simulink model "EKF_SIL_02_newdelIpsOOSM"  (R2015a)
settings: Solver=ode45  StartTime=0.0  StopTime=50  RelTol=1e-3
model workspace: external: MATLAB File InitOOSM.m (data not in the file)
values from neighbouring files (symbols this model uses):
  Cov_nu = [0.005 0 0 0 ... (first row only)    [InitOOSM.m]    (also in InitSIL.m; Init_Model_02_Simulink.m; Init_Model_02_Simulink_SIL1.m)
  Cov_r = [0.003 0 0 ... (first row only)    [InitOOSM.m]    (also in InitSIL.m; Init_Model_02_Simulink.m; Init_Model_02_Simulink_SIL1.m)
  e_force_x = 0    [InitOOSM.m]    (also in InitSIL.m; Init_Model_02_Simulink.m; Init_Model_02_Simulink_SIL1.m)
  e_force_y = 0    [InitOOSM.m]    (also in InitSIL.m; Init_Model_02_Simulink.m; Init_Model_02_Simulink_SIL1.m)
  e_force_z = 0    [InitOOSM.m]    (also in InitSIL.m; Init_Model_02_Simulink.m; Init_Model_02_Simulink_SIL1.m)
  ieps = [-0.7071;0;0;0.7071]    [InitOOSM.m]    (also in InitSIL.m; Init_Model_02_Simulink.m = [-0.7071; 0; 0; 0.7071]; Init_Model_02_Simulink_SIL1.m)
  ita = [0.5;0.5;0.5;0.5]    [InitOOSM.m]    (also in InitSIL.m; Init_Model_02_Simulink.m = [0.5; 0.5; 0.5; 0.5]; Init_Model_02_Simulink_SIL1.m)
  n = 0.00    (= 0)    [InitOOSM.m]    (also in InitSIL.m; Init_Model_02_Simulink.m; Init_Model_02_Simulink_SIL1.m)
  P_0 = 0.5*eye(18,18)    [InitOOSM.m]    (also in InitSIL.m = 0.05*eye(12,12); Init_Model_02_Simulink.m = 0.005*eye(12,12); Init_Model_02_Simulink_SIL1.m = 0.005*eye(12,12))
  P_k = Simulink.Signal    [InitOOSM.m]    (also in InitSIL.m; Init_Model_02_Simulink.m; Init_Model_02_Simulink_SIL1.m)
  p_x = 0.75    [InitOOSM.m]    (also in InitSIL.m; Init_Model_02_Simulink.m; Init_Model_02_Simulink_SIL1.m)
  p_y = 0.125    [InitOOSM.m]    (also in InitSIL.m; Init_Model_02_Simulink.m; Init_Model_02_Simulink_SIL1.m)
  p_z = -0.8    [InitOOSM.m]    (also in InitSIL.m; Init_Model_02_Simulink.m; Init_Model_02_Simulink_SIL1.m)
  parameter_gravitation = 3.986005E+14    (= 398600500000000)    [InitOOSM.m]    (also in InitSIL.m; Init_Model_02_Simulink.m; Init_Model_02_Simulink_SIL1.m)
  rho = [0.04;0;0.3]    [InitOOSM.m]    (also in InitSIL.m; Init_Model_02_Simulink.m = [0.04; 0; 0.3]; Init_Model_02_Simulink_SIL1.m)
  rho_c = [-0.00017;   -0.9780;   -0.1854]    [InitOOSM.m]    (also in InitSIL.m = [0.00036;   -0.9865;   -0.1854]; Init_Model_02_Simulink.m = [0.00036; -0.9865; -0.1854]; Init_Model_02_Simulink_SIL1.m = [0.00036;   -0.9865;   -0.1854])
  sig_f = 2E-6    (= 2e-06)    [InitOOSM.m]    (also in InitSIL.m; Init_Model_02_Simulink.m; Init_Model_02_Simulink_SIL1.m)
  sig_tau = 2.5E-5    (= 2.5e-05)    [InitOOSM.m]    (also in InitSIL.m; Init_Model_02_Simulink.m; Init_Model_02_Simulink_SIL1.m)
  t_delta = 0.2    [InitOOSM.m]    (also in InitSIL.m; Init_Model_02_Simulink.m; Init_Model_02_Simulink_SIL1.m)
  t_Kalman = 0.01    [InitOOSM.m]    (also in InitSIL.m; Init_Model_02_Simulink.m; Init_Model_02_Simulink_SIL1.m)
  t_RobotSense = 0.05    [InitOOSM.m]    (also in InitSIL.m; Init_Model_02_Simulink.m; Init_Model_02_Simulink_SIL1.m)
  tau_1 = 0    [InitOOSM.m]    (also in InitSIL.m; Init_Model_02_Simulink.m; Init_Model_02_Simulink_SIL1.m)
  tau_2 = 0    [InitOOSM.m]    (also in InitSIL.m; Init_Model_02_Simulink.m; Init_Model_02_Simulink_SIL1.m)
  tau_3 = 0    [InitOOSM.m]    (also in InitSIL.m; Init_Model_02_Simulink.m; Init_Model_02_Simulink_SIL1.m)
  U_n_d = Simulink.Signal    [InitOOSM.m]    (also in InitSIL.m; Init_Model_02_Simulink.m; Init_Model_02_Simulink_SIL1.m)
  X_a_0 = [0; 0; 0; 1; 0; 0; 0; 0; 0; 0; 0; 0; 0;0;0;0;0;0;0;1]    [InitOOSM.m]    (also in InitSIL.m = [0; 0; 0; 1; 0; 0; 0; 0; 0; 0; 0; 0; 0]; Init_Model_02_Simulink.m = [0;0;0;0.707000000000000;0.707000000000000;0.200000000000000; Init_Model_02_Simulink_SIL1.m = [0;0;0.707;0.707;0.2;-0.02;0.0001;0.02;-1.80;0.50;-0.05;0.00)
  x_k = Simulink.Signal    [InitOOSM.m]    (also in InitSIL.m; Init_Model_02_Simulink.m; Init_Model_02_Simulink_SIL1.m)
libraries: simulink x9, dspmtrx3 x4, aerolibtransform2 x2, visionsinks x1
(part 5 of 6)

== system EKF_SIL_02_newdelIpsOOSM/EKF/Measurement Update/Update with K(k) and predict current state/Create H_k/Create Skew Symmetric1/Create 3x3 matrix ==
  a11 : Inport
  a12 : Inport  Port=2
  a13 : Inport  Port=3
  a21 : Inport  Port=4
  a22 : Inport  Port=5
  a23 : Inport  Port=6
  a31 : Inport  Port=7
  a32 : Inport  Port=8
  a33 : Inport  Port=9
  Math Function : Math  Operator=transpose  SaturateOnIntegerOverflow=on
  Reshape (9) to [3x3] column-major : Reshape  OutputDimensionality=Customize  OutputDimensions=[3,3]
  Vector Concatenate : Concatenate  NumInputs=9
  Matrix : Outport
  wires:
  Math Function/1 -> Matrix/1
  Reshape (9) to [3x3] column-major/1 -> Math Function/1
  a21/1 -> Vector Concatenate/4
  a32/1 -> Vector Concatenate/8
  a31/1 -> Vector Concatenate/7
  a23/1 -> Vector Concatenate/6
  a13/1 -> Vector Concatenate/3
  a12/1 -> Vector Concatenate/2
  a11/1 -> Vector Concatenate/1
  Vector Concatenate/1 -> Reshape (9) to [3x3] column-major/1
  a22/1 -> Vector Concatenate/5
  a33/1 -> Vector Concatenate/9

== system EKF_SIL_02_newdelIpsOOSM/EKF/Measurement Update/Update with K(k) and predict current state/Create H_k/Create Skew Symmetric2/Create 3x3 matrix ==
  a11 : Inport
  a12 : Inport  Port=2
  a13 : Inport  Port=3
  a21 : Inport  Port=4
  a22 : Inport  Port=5
  a23 : Inport  Port=6
  a31 : Inport  Port=7
  a32 : Inport  Port=8
  a33 : Inport  Port=9
  Math Function : Math  Operator=transpose  SaturateOnIntegerOverflow=on
  Reshape (9) to [3x3] column-major : Reshape  OutputDimensionality=Customize  OutputDimensions=[3,3]
  Vector Concatenate : Concatenate  NumInputs=9
  Matrix : Outport
  wires:
  a33/1 -> Vector Concatenate/9
  a22/1 -> Vector Concatenate/5
  Vector Concatenate/1 -> Reshape (9) to [3x3] column-major/1
  a11/1 -> Vector Concatenate/1
  a12/1 -> Vector Concatenate/2
  a13/1 -> Vector Concatenate/3
  a23/1 -> Vector Concatenate/6
  a31/1 -> Vector Concatenate/7
  a32/1 -> Vector Concatenate/8
  a21/1 -> Vector Concatenate/4
  Reshape (9) to [3x3] column-major/1 -> Math Function/1
  Math Function/1 -> Matrix/1

== system EKF_SIL_02_newdelIpsOOSM/EKF/Measurement Update/Update with K(k) and predict current state/Create H_k/Create Skew Symmetric3/Create 3x3 matrix ==
  a11 : Inport
  a12 : Inport  Port=2
  a13 : Inport  Port=3
  a21 : Inport  Port=4
  a22 : Inport  Port=5
  a23 : Inport  Port=6
  a31 : Inport  Port=7
  a32 : Inport  Port=8
  a33 : Inport  Port=9
  Math Function : Math  Operator=transpose  SaturateOnIntegerOverflow=on
  Reshape (9) to [3x3] column-major : Reshape  OutputDimensionality=Customize  OutputDimensions=[3,3]
  Vector Concatenate : Concatenate  NumInputs=9
  Matrix : Outport
  wires:
  a33/1 -> Vector Concatenate/9
  a22/1 -> Vector Concatenate/5
  Vector Concatenate/1 -> Reshape (9) to [3x3] column-major/1
  a11/1 -> Vector Concatenate/1
  a12/1 -> Vector Concatenate/2
  a13/1 -> Vector Concatenate/3
  a23/1 -> Vector Concatenate/6
  a31/1 -> Vector Concatenate/7
  a32/1 -> Vector Concatenate/8
  a21/1 -> Vector Concatenate/4
  Reshape (9) to [3x3] column-major/1 -> Math Function/1
  Math Function/1 -> Matrix/1

== system EKF_SIL_02_newdelIpsOOSM/EKF/Measurement Update/Update with K(k) and predict current state/Create H_k/Subsystem/norm  ==
  vector : Inport
  Dot Product : DotProduct  InputSameDT=on  OutDataTypeStr=Inherit: Inherit via internal rule
  "norm " : Outport
  wires:
  vector/1 -> Dot Product/2, Dot Product/1
  Dot Product/1 -> "norm "/1

== system EKF_SIL_02_newdelIpsOOSM/EKF/Measurement Update/Update with K(k) and predict current state/Create H_k/Subsystem1/norm  ==
  vector : Inport
  Dot Product : DotProduct  InputSameDT=on  OutDataTypeStr=Inherit: Inherit via internal rule
  "norm " : Outport
  wires:
  Dot Product/1 -> "norm "/1
  vector/1 -> Dot Product/1, Dot Product/2

== system EKF_SIL_02_newdelIpsOOSM/EKF/Measurement Update/Update with K(k) and predict current state/Create X_a from X/Create q_nominal /norm  ==
  vector : Inport
  Dot Product : DotProduct  InputSameDT=on  OutDataTypeStr=Inherit: Inherit via internal rule
  "norm " : Outport
  wires:
  vector/1 -> Dot Product/2, Dot Product/1
  Dot Product/1 -> "norm "/1

== system EKF_SIL_02_newdelIpsOOSM/EKF/Measurement Update/Update with K(k) and predict current state/Create X_a from X/Create q_nominal 1/norm  ==
  vector : Inport
  Dot Product : DotProduct  InputSameDT=on  OutDataTypeStr=Inherit: Inherit via internal rule
  "norm " : Outport
  wires:
  vector/1 -> Dot Product/2, Dot Product/1
  Dot Product/1 -> "norm "/1

== system EKF_SIL_02_newdelIpsOOSM/EKF/Measurement Update/Update with K(k) and predict current state/Create h/Create Rotation Matrix /Create Skew Symmetric ==
  vector : Inport
  0 : Constant  Value=0
  Create 3x3 matrix : Subsystem
  Demux : Demux  Outputs=3
  Demux1 : Demux  Outputs=3
  Gain : Gain  Gain=-1
  skew symmetric Matrix : Outport
  wires:
  0/1 -> Create 3x3 matrix/1(a11), Create 3x3 matrix/9(a33), Create 3x3 matrix/5(a22)
  Demux/3 -> Create 3x3 matrix/2(a12)
  Demux1/2 -> Create 3x3 matrix/3(a13)
  Demux1/3 -> Create 3x3 matrix/4(a21)
  Demux/1 -> Create 3x3 matrix/6(a23)
  vector/1 -> Demux1/1, Gain/1
  Create 3x3 matrix/1(Matrix) -> skew symmetric Matrix/1
  Gain/1 -> Demux/1
  Demux/2 -> Create 3x3 matrix/7(a31)
  Demux1/1 -> Create 3x3 matrix/8(a32)

== system EKF_SIL_02_newdelIpsOOSM/EKF/Measurement Update/Update with K(k) and predict current state/Create h/Create Rotation Matrix 1/Create Skew Symmetric ==
  vector : Inport
  0 : Constant  Value=0
  Create 3x3 matrix : Subsystem
  Demux : Demux  Outputs=3
  Demux1 : Demux  Outputs=3
  Gain : Gain  Gain=-1
  skew symmetric Matrix : Outport
  wires:
  0/1 -> Create 3x3 matrix/1(a11), Create 3x3 matrix/9(a33), Create 3x3 matrix/5(a22)
  Demux/3 -> Create 3x3 matrix/2(a12)
  Demux1/2 -> Create 3x3 matrix/3(a13)
  Demux1/3 -> Create 3x3 matrix/4(a21)
  Demux/1 -> Create 3x3 matrix/6(a23)
  vector/1 -> Demux1/1, Gain/1
  Create 3x3 matrix/1(Matrix) -> skew symmetric Matrix/1
  Gain/1 -> Demux/1
  Demux/2 -> Create 3x3 matrix/7(a31)
  Demux1/1 -> Create 3x3 matrix/8(a32)

== system EKF_SIL_02_newdelIpsOOSM/EKF/Measurement Update/Update with K(k) and predict current state/Create h/Create Rotation Matrix 2/Create Skew Symmetric ==
  vector : Inport
  0 : Constant  Value=0
  Create 3x3 matrix : Subsystem
  Demux : Demux  Outputs=3
  Demux1 : Demux  Outputs=3
  Gain : Gain  Gain=-1
  skew symmetric Matrix : Outport
  wires:
  Demux1/1 -> Create 3x3 matrix/8(a32)
  Demux/2 -> Create 3x3 matrix/7(a31)
  Gain/1 -> Demux/1
  Create 3x3 matrix/1(Matrix) -> skew symmetric Matrix/1
  vector/1 -> Gain/1, Demux1/1
  Demux/1 -> Create 3x3 matrix/6(a23)
  Demux1/3 -> Create 3x3 matrix/4(a21)
  Demux1/2 -> Create 3x3 matrix/3(a13)
  Demux/3 -> Create 3x3 matrix/2(a12)
  0/1 -> Create 3x3 matrix/5(a22), Create 3x3 matrix/9(a33), Create 3x3 matrix/1(a11)

== system EKF_SIL_02_newdelIpsOOSM/EKF/Measurement Update/Update with K(k) and predict current state/Create h/Subsystem/norm  ==
  vector : Inport
  Dot Product : DotProduct  InputSameDT=on  OutDataTypeStr=Inherit: Inherit via internal rule
  "norm " : Outport
  wires:
  vector/1 -> Dot Product/2, Dot Product/1
  Dot Product/1 -> "norm "/1

== system EKF_SIL_02_newdelIpsOOSM/EKF/Measurement Update/Update with K(k) and predict current state/Create h/Subsystem1/norm  ==
  vector : Inport
  Dot Product : DotProduct  InputSameDT=on  OutDataTypeStr=Inherit: Inherit via internal rule
  "norm " : Outport
  wires:
  Dot Product/1 -> "norm "/1
  vector/1 -> Dot Product/1, Dot Product/2

== system EKF_SIL_02_newdelIpsOOSM/EKF/Measurement Update/Update with K(k) and predict current state/Create h/Subsystem2/norm  ==
  vector : Inport
  Dot Product : DotProduct  InputSameDT=on  OutDataTypeStr=Inherit: Inherit via internal rule
  "norm " : Outport
  wires:
  vector/1 -> Dot Product/2, Dot Product/1
  Dot Product/1 -> "norm "/1

== system EKF_SIL_02_newdelIpsOOSM/EKF/Measurement Update/Update with K(k) and predict current state/Create h/Subsystem3/norm  ==
  vector : Inport
  Dot Product : DotProduct  InputSameDT=on  OutDataTypeStr=Inherit: Inherit via internal rule
  "norm " : Outport
  wires:
  Dot Product/1 -> "norm "/1
  vector/1 -> Dot Product/1, Dot Product/2

== system EKF_SIL_02_newdelIpsOOSM/EKF/OOSM_KF/OOSM_KF/Create X from X_a1/Create del_q [body]/q_star ==
  q : Inport
  Demux : Demux
  Mux : Mux  Inputs=3
  Mux1 : Mux  Inputs=2
  Unary Minus : UnaryMinus
  q_star : Outport
  wires:
  Unary Minus/1 -> Mux1/1
  Demux/2 -> Mux/2
  Mux/1 -> Unary Minus/1
  Demux/4 -> Mux1/2
  Demux/3 -> Mux/3
  q/1 -> Demux/1
  Demux/1 -> Mux/1
  Mux1/1 -> q_star/1

== system EKF_SIL_02_newdelIpsOOSM/EKF/OOSM_KF/OOSM_KF/Create X from X_a1/Create del_q [inertial]/q_star ==
  q : Inport
  Demux : Demux
  Mux : Mux  Inputs=3
  Mux1 : Mux  Inputs=2
  Unary Minus : UnaryMinus
  q_star : Outport
  wires:
  Unary Minus/1 -> Mux1/1
  Demux/2 -> Mux/2
  Mux/1 -> Unary Minus/1
  Demux/4 -> Mux1/2
  Demux/3 -> Mux/3
  q/1 -> Demux/1
  Demux/1 -> Mux/1
  Mux1/1 -> q_star/1

== system EKF_SIL_02_newdelIpsOOSM/EKF/OOSM_KF/OOSM_KF/State Propagation/Create M/Create 3x3 matrix ==
  a11 : Inport
  a12 : Inport  Port=2
  a13 : Inport  Port=3
  a21 : Inport  Port=4
  a22 : Inport  Port=5
  a23 : Inport  Port=6
  a31 : Inport  Port=7
  a32 : Inport  Port=8
  a33 : Inport  Port=9
  Math Function : Math  Operator=transpose  SaturateOnIntegerOverflow=on
  Reshape (9) to [3x3] column-major : Reshape  OutputDimensionality=Customize  OutputDimensions=[3,3]
  Vector Concatenate : Concatenate  NumInputs=9
  Matrix : Outport
  wires:
  a33/1 -> Vector Concatenate/9
  a22/1 -> Vector Concatenate/5
  Vector Concatenate/1 -> Reshape (9) to [3x3] column-major/1
  a11/1 -> Vector Concatenate/1
  a12/1 -> Vector Concatenate/2
  a13/1 -> Vector Concatenate/3
  a23/1 -> Vector Concatenate/6
  a31/1 -> Vector Concatenate/7
  a32/1 -> Vector Concatenate/8
  a21/1 -> Vector Concatenate/4
  Reshape (9) to [3x3] column-major/1 -> Math Function/1
  Math Function/1 -> Matrix/1

== system EKF_SIL_02_newdelIpsOOSM/EKF/OOSM_KF/OOSM_KF/State Propagation/Create Rotation Matrix 1/Create Skew Symmetric ==
  vector : Inport
  0 : Constant  Value=0
  Create 3x3 matrix : Subsystem
  Demux : Demux  Outputs=3
  Demux1 : Demux  Outputs=3
  Gain : Gain  Gain=-1
  skew symmetric Matrix : Outport
  wires:
  0/1 -> Create 3x3 matrix/1(a11), Create 3x3 matrix/9(a33), Create 3x3 matrix/5(a22)
  Demux/3 -> Create 3x3 matrix/2(a12)
  Demux1/2 -> Create 3x3 matrix/3(a13)
  Demux1/3 -> Create 3x3 matrix/4(a21)
  Demux/1 -> Create 3x3 matrix/6(a23)
  vector/1 -> Demux1/1, Gain/1
  Create 3x3 matrix/1(Matrix) -> skew symmetric Matrix/1
  Gain/1 -> Demux/1
  Demux/2 -> Create 3x3 matrix/7(a31)
  Demux1/1 -> Create 3x3 matrix/8(a32)

== system EKF_SIL_02_newdelIpsOOSM/EKF/OOSM_KF/OOSM_enable/Enabled Subsystem/Create H_k/Create Rotation Matrix  ==
  q : Inport
  Add : Sum
  Add5 : Sum  Inputs=+++
  Constant1 : Constant  Value=-1
  Create Skew Symmetric : Subsystem
  Gain : Gain  Gain=2
  Gain1 : Gain  Gain=2
  Gain2 : Gain  Gain=2
  I : Constant  Value=eye(3,3)
  Math Function : Math  Operator=square  SaturateOnIntegerOverflow=on
  Math Function1 : Math  Operator=transpose  SaturateOnIntegerOverflow=on
  Product1 : Product
  Product2 : Product
  Product3 : Product  Multiplication=Matrix(*)
  Selector2 : Selector  NumberOfDimensions=2  InputPortWidth=3  IndexOptions=Index vector (dialog),Index vector (dialog)  Indices=[1 2 3],1  OutputSizes=1,1
  Selector3 : Selector  NumberOfDimensions=2  InputPortWidth=3  IndexOptions=Index vector (dialog),Index vector (dialog)  Indices=[4],1  OutputSizes=1,1
  R : Outport
  wires:
  Gain/1 -> Add/1
  Math Function/1 -> Gain/1
  Constant1/1 -> Add/2
  Selector3/1 -> Product2/2, Math Function/1
  Add/1 -> Product1/1
  I/1 -> Product1/2
  Selector2/1 -> Math Function1/1, Product3/1, Create Skew Symmetric/1(vector)
  Gain2/1 -> Add5/1
  Product2/1 -> Add5/2
  Create Skew Symmetric/1(skew symmetric Matrix) -> Gain1/1
  Gain1/1 -> Product2/1
  Product1/1 -> Add5/3
  Math Function1/1 -> Product3/2
  Product3/1 -> Gain2/1
  Add5/1 -> R/1
  q/1 -> Selector3/1, Selector2/1

== system EKF_SIL_02_newdelIpsOOSM/EKF/OOSM_KF/OOSM_enable/Enabled Subsystem/Create H_k/Create Skew Symmetric ==
  vector : Inport
  0 : Constant  Value=0
  Create 3x3 matrix : Subsystem
  Demux : Demux  Outputs=3
  Demux1 : Demux  Outputs=3
  Gain : Gain  Gain=-1
  skew symmetric Matrix : Outport
  wires:
  0/1 -> Create 3x3 matrix/1(a11), Create 3x3 matrix/9(a33), Create 3x3 matrix/5(a22)
  Demux/3 -> Create 3x3 matrix/2(a12)
  Demux1/2 -> Create 3x3 matrix/3(a13)
  Demux1/3 -> Create 3x3 matrix/4(a21)
  Demux/1 -> Create 3x3 matrix/6(a23)
  vector/1 -> Demux1/1, Gain/1
  Create 3x3 matrix/1(Matrix) -> skew symmetric Matrix/1
  Gain/1 -> Demux/1
  Demux/2 -> Create 3x3 matrix/7(a31)
  Demux1/1 -> Create 3x3 matrix/8(a32)

== system EKF_SIL_02_newdelIpsOOSM/EKF/OOSM_KF/Subsystem/Dynamic Model (Differential equations)2/Dynamic Model (Differential equations)/Orbital Dynamics  ==
  r : Inport
  Mu : Inport  Port=2
  n : Inport  Port=3
  "r_dot " : Inport  Port=4
  " " : Constant  Value=[0;0]  SampleTime=-1
  Add : Sum
  Create Skew Symmetric : Subsystem
  Divide : Product  Inputs=*/
  Divide1 : Product  Inputs=*/
  Fcn : Fcn  Expr=u(1)^3
  Fcn1 : Fcn  Expr=u(1)^(1/3)
  Gain : Gain  Gain=-2
  Product : Product  Multiplication=Matrix(*)
  Product1 : Product  Multiplication=Matrix(*)
  Product2 : Product  Multiplication=Matrix(*)
  Product3 : Product
  Product4 : Product
  Product5 : Product
  Sum : Sum  Inputs=+--++
  Vector Concatenate1 : Concatenate
  "conc_re " : Constant  Value=[0;0]  SampleTime=-1
  "e_force " : Constant  Value=[e_force_x;e_force_y;e_force_z]  SampleTime=-1
  "norm " : Subsystem
  re : Concatenate
  "r_ddot " : Outport
  wires:
  Sum/1 -> "r_ddot "/1
  "e_force "/1 -> Sum/5
  Divide/1 -> Fcn1/1
  Fcn/1 -> Divide1/2
  Fcn1/1 -> re/1
  Divide1/1 -> Sum/3
  "r_dot "/1 -> Product/2
  Product4/1 -> Sum/4
  r/1 -> Add/1, Product1/2
  Product2/1 -> Sum/2
  Gain/1 -> Sum/1
  Add/1 -> Product5/2, "norm "/1(vector)
  Vector Concatenate1/1 -> Create Skew Symmetric/1(vector)
  Product3/1 -> Product4/2, Divide/2
  n/1 -> Product3/1, Vector Concatenate1/2, Product3/2
  "norm "/1("norm ") -> Fcn/1
  Product5/1 -> Divide1/1
  re/1 -> Add/2, Product4/1
  "conc_re "/1 -> re/2
  Product/1 -> Gain/1
  Mu/1 -> Divide/1, Product5/1
  Product1/1 -> Product2/2
  Create Skew Symmetric/1(skew symmetric Matrix) -> Product2/1, Product1/1, Product/1
  " "/1 -> Vector Concatenate1/1

== system EKF_SIL_02_newdelIpsOOSM/EKF/OOSM_KF/Subsystem/Dynamic Model (Differential equations)2/Dynamic Model (Differential equations)/Pose Servicer base//EE ==
  V : Inport
  rho_c : Inport  Port=2
  "ieps " : Inport  Port=3
  0 : Constant  Value=0  SampleTime=-1
  Create Skew Symmetric : Subsystem
  Display : Display
  Display1 : Display
  Gain : Gain  Gain=0.5
  MATLAB Function1 : MATLAB Function  TreatAsAtomicUnit=on
  Mux : Mux  Inputs=2
  Selector : Selector  InputPortWidth=6  Indices=[1:3]
  Selector1 : Selector  InputPortWidth=6  Indices=[4:6]
  Sum : Sum  Inputs=|++
  flag : Constant  Value=0  SampleTime=-1
  "mult " : Product  Multiplication=Matrix(*)
  mult 1 : Product  Multiplication=Matrix(*)
  rho_c_dot : Outport
  ieps_dot : Outport  Port=2
  wires:
  flag/1 -> MATLAB Function1/2(flag)
  0/1 -> Mux/2
  MATLAB Function1/1(CrossTensor) -> "mult "/1
  Mux/1 -> "mult "/2
  "mult "/1 -> Gain/1
  V/1 -> Selector1/1, Display1/1, Selector/1
  Selector/1 -> Sum/2
  Selector1/1 -> Mux/1, Create Skew Symmetric/1(vector)
  Create Skew Symmetric/1(skew symmetric Matrix) -> mult 1/1
  rho_c/1 -> mult 1/2
  mult 1/1 -> Sum/1
  Sum/1 -> Display/1, rho_c_dot/1
  "ieps "/1 -> MATLAB Function1/1(q)
  Gain/1 -> ieps_dot/1

== system EKF_SIL_02_newdelIpsOOSM/EKF/OOSM_KF/Subsystem/Dynamic Model (Differential equations)2/Dynamic Model (Differential equations)/Quaternion Kinematics ==
  q : Inport
  omega_rel : Inport  Port=2
  Constant2 : Constant  Value=0.5  SampleTime=-1
  MATLAB Function : MATLAB Function  TreatAsAtomicUnit=on
  Product : Product  Multiplication=Matrix(*)
  Product1 : Product
  flag : Constant  SampleTime=-1
  q_dot : Outport
  wires:
  Product/1 -> Product1/1
  Product1/1 -> q_dot/1
  omega_rel/1 -> Product/2
  q/1 -> MATLAB Function/1(q)
  Constant2/1 -> Product1/2
  flag/1 -> MATLAB Function/2(flag)
  MATLAB Function/1(CrossTensor) -> Product/1

== system EKF_SIL_02_newdelIpsOOSM/EKF/OOSM_KF/Subsystem/Dynamic Model (Differential equations)2/Dynamic Model (Differential equations)/Rotational Dynamics ==
  omega : Inport
  p : Inport  Port=2
  Add : Sum
  Create  J : Subsystem
  Create Psi : Subsystem
  Product : Product  Multiplication=Matrix(*)
  tau : Constant  Value=[tau_1;tau_2;tau_3]  SampleTime=-1
  omega_dot : Outport
  wires:
  tau/1 -> Product/2
  Create  J/1("J_k ") -> Product/1
  p/1 -> Create  J/1(p), Create Psi/2(p)
  Product/1 -> Add/2
  Add/1 -> omega_dot/1
  Create Psi/1(Psi) -> Add/1
  omega/1 -> Create Psi/1("omega ")

== system EKF_SIL_02_newdelIpsOOSM/EKF/Predictor/Create State error covariance (P)/State Propagation/Create M/Create 3x3 matrix ==
  a11 : Inport
  a12 : Inport  Port=2
  a13 : Inport  Port=3
  a21 : Inport  Port=4
  a22 : Inport  Port=5
  a23 : Inport  Port=6
  a31 : Inport  Port=7
  a32 : Inport  Port=8
  a33 : Inport  Port=9
  Math Function : Math  Operator=transpose  SaturateOnIntegerOverflow=on
  Reshape (9) to [3x3] column-major : Reshape  OutputDimensionality=Customize  OutputDimensions=[3,3]
  Vector Concatenate : Concatenate  NumInputs=9
  Matrix : Outport
  wires:
  a33/1 -> Vector Concatenate/9
  a22/1 -> Vector Concatenate/5
  Vector Concatenate/1 -> Reshape (9) to [3x3] column-major/1
  a11/1 -> Vector Concatenate/1
  a12/1 -> Vector Concatenate/2
  a13/1 -> Vector Concatenate/3
  a23/1 -> Vector Concatenate/6
  a31/1 -> Vector Concatenate/7
  a32/1 -> Vector Concatenate/8
  a21/1 -> Vector Concatenate/4
  Reshape (9) to [3x3] column-major/1 -> Math Function/1
  Math Function/1 -> Matrix/1

== system EKF_SIL_02_newdelIpsOOSM/EKF/Predictor/Create State error covariance (P)/State Propagation/Create Rotation Matrix 1/Create Skew Symmetric ==
  vector : Inport
  0 : Constant  Value=0
  Create 3x3 matrix : Subsystem
  Demux : Demux  Outputs=3
  Demux1 : Demux  Outputs=3
  Gain : Gain  Gain=-1
  skew symmetric Matrix : Outport
  wires:
  0/1 -> Create 3x3 matrix/1(a11), Create 3x3 matrix/9(a33), Create 3x3 matrix/5(a22)
  Demux/3 -> Create 3x3 matrix/2(a12)
  Demux1/2 -> Create 3x3 matrix/3(a13)
  Demux1/3 -> Create 3x3 matrix/4(a21)
  Demux/1 -> Create 3x3 matrix/6(a23)
  vector/1 -> Demux1/1, Gain/1
  Create 3x3 matrix/1(Matrix) -> skew symmetric Matrix/1
  Gain/1 -> Demux/1
  Demux/2 -> Create 3x3 matrix/7(a31)
  Demux1/1 -> Create 3x3 matrix/8(a32)

== system EKF_SIL_02_newdelIpsOOSM/EKF/Predictor/Integrator/Dynamic Model (Differential equations)2/Dynamic Model (Differential equations)/Orbital Dynamics  ==
  r : Inport
  Mu : Inport  Port=2
  n : Inport  Port=3
  "r_dot " : Inport  Port=4
  " " : Constant  Value=[0;0]  SampleTime=-1
  Add : Sum
  Create Skew Symmetric : Subsystem
  Divide : Product  Inputs=*/
  Divide1 : Product  Inputs=*/
  Fcn : Fcn  Expr=u(1)^3
  Fcn1 : Fcn  Expr=u(1)^(1/3)
  Gain : Gain  Gain=-2
  Product : Product  Multiplication=Matrix(*)
  Product1 : Product  Multiplication=Matrix(*)
  Product2 : Product  Multiplication=Matrix(*)
  Product3 : Product
  Product4 : Product
  Product5 : Product
  Sum : Sum  Inputs=+--++
  Vector Concatenate1 : Concatenate
  "conc_re " : Constant  Value=[0;0]  SampleTime=-1
  "e_force " : Constant  Value=[e_force_x;e_force_y;e_force_z]  SampleTime=-1
  "norm " : Subsystem
  re : Concatenate
  "r_ddot " : Outport
  wires:
  Sum/1 -> "r_ddot "/1
  "e_force "/1 -> Sum/5
  Divide/1 -> Fcn1/1
  Fcn/1 -> Divide1/2
  Fcn1/1 -> re/1
  Divide1/1 -> Sum/3
  "r_dot "/1 -> Product/2
  Product4/1 -> Sum/4
  r/1 -> Add/1, Product1/2
  Product2/1 -> Sum/2
  Gain/1 -> Sum/1
  Add/1 -> Product5/2, "norm "/1(vector)
  Vector Concatenate1/1 -> Create Skew Symmetric/1(vector)
  Product3/1 -> Product4/2, Divide/2
  n/1 -> Product3/1, Vector Concatenate1/2, Product3/2
  "norm "/1("norm ") -> Fcn/1
  Product5/1 -> Divide1/1
  re/1 -> Add/2, Product4/1
  "conc_re "/1 -> re/2
  Product/1 -> Gain/1
  Mu/1 -> Divide/1, Product5/1
  Product1/1 -> Product2/2
  Create Skew Symmetric/1(skew symmetric Matrix) -> Product2/1, Product1/1, Product/1
  " "/1 -> Vector Concatenate1/1

== system EKF_SIL_02_newdelIpsOOSM/EKF/Predictor/Integrator/Dynamic Model (Differential equations)2/Dynamic Model (Differential equations)/Pose Servicer base//EE ==
  V : Inport
  rho_c : Inport  Port=2
  "ieps " : Inport  Port=3
  0 : Constant  Value=0  SampleTime=-1
  Create Skew Symmetric : Subsystem
  Display : Display
  Display1 : Display
  Gain : Gain  Gain=0.5
  MATLAB Function1 : MATLAB Function  TreatAsAtomicUnit=on
  Mux : Mux  Inputs=2
  Selector : Selector  InputPortWidth=6  Indices=[1:3]
  Selector1 : Selector  InputPortWidth=6  Indices=[4:6]
  Sum : Sum  Inputs=|++
  flag : Constant  Value=0  SampleTime=-1
  "mult " : Product  Multiplication=Matrix(*)
  mult 1 : Product  Multiplication=Matrix(*)
  rho_c_dot : Outport
  ieps_dot : Outport  Port=2
  wires:
  flag/1 -> MATLAB Function1/2(flag)
  0/1 -> Mux/2
  MATLAB Function1/1(CrossTensor) -> "mult "/1
  Mux/1 -> "mult "/2
  "mult "/1 -> Gain/1
  V/1 -> Selector1/1, Display1/1, Selector/1
  Selector/1 -> Sum/2
  Selector1/1 -> Mux/1, Create Skew Symmetric/1(vector)
  Create Skew Symmetric/1(skew symmetric Matrix) -> mult 1/1
  rho_c/1 -> mult 1/2
  mult 1/1 -> Sum/1
  Sum/1 -> Display/1, rho_c_dot/1
  "ieps "/1 -> MATLAB Function1/1(q)
  Gain/1 -> ieps_dot/1

== system EKF_SIL_02_newdelIpsOOSM/EKF/Predictor/Integrator/Dynamic Model (Differential equations)2/Dynamic Model (Differential equations)/Quaternion Kinematics ==
  q : Inport
  omega_rel : Inport  Port=2
  Constant2 : Constant  Value=0.5  SampleTime=-1
  MATLAB Function : MATLAB Function  TreatAsAtomicUnit=on
  Product : Product  Multiplication=Matrix(*)
  Product1 : Product
  flag : Constant  SampleTime=-1
  q_dot : Outport
  wires:
  Product/1 -> Product1/1
  Product1/1 -> q_dot/1
  omega_rel/1 -> Product/2
  q/1 -> MATLAB Function/1(q)
  Constant2/1 -> Product1/2
  flag/1 -> MATLAB Function/2(flag)
  MATLAB Function/1(CrossTensor) -> Product/1

== system EKF_SIL_02_newdelIpsOOSM/EKF/Predictor/Integrator/Dynamic Model (Differential equations)2/Dynamic Model (Differential equations)/Rotational Dynamics ==
  omega : Inport
  p : Inport  Port=2
  Add : Sum
  Create  J : Subsystem
  Create Psi : Subsystem
  Product : Product  Multiplication=Matrix(*)
  tau : Constant  Value=[tau_1;tau_2;tau_3]  SampleTime=-1
  omega_dot : Outport
  wires:
  tau/1 -> Product/2
  Create  J/1("J_k ") -> Product/1
  p/1 -> Create  J/1(p), Create Psi/2(p)
  Product/1 -> Add/2
  Add/1 -> omega_dot/1
  Create Psi/1(Psi) -> Add/1
  omega/1 -> Create Psi/1("omega ")

== system EKF_SIL_02_newdelIpsOOSM/Plots and display/Create Measurements [Pose]1/Create Measurements [Position]/Create Rotation Matrix /Create Skew Symmetric/Create 3x3 matrix ==
  a11 : Inport
  a12 : Inport  Port=2
  a13 : Inport  Port=3
  a21 : Inport  Port=4
  a22 : Inport  Port=5
  a23 : Inport  Port=6
  a31 : Inport  Port=7
  a32 : Inport  Port=8
  a33 : Inport  Port=9
  Math Function : Math  Operator=transpose  SaturateOnIntegerOverflow=on
  Reshape (9) to [3x3] column-major : Reshape  OutputDimensionality=Customize  OutputDimensions=[3,3]
  Vector Concatenate : Concatenate  NumInputs=9
  Matrix : Outport
  wires:
  a33/1 -> Vector Concatenate/9
  a22/1 -> Vector Concatenate/5
  Vector Concatenate/1 -> Reshape (9) to [3x3] column-major/1
  a11/1 -> Vector Concatenate/1
  a12/1 -> Vector Concatenate/2
  a13/1 -> Vector Concatenate/3
  a23/1 -> Vector Concatenate/6
  a31/1 -> Vector Concatenate/7
  a32/1 -> Vector Concatenate/8
  a21/1 -> Vector Concatenate/4
  Reshape (9) to [3x3] column-major/1 -> Math Function/1
  Math Function/1 -> Matrix/1

== system EKF_SIL_02_newdelIpsOOSM/Plots and display/Create Measurements [Pose]2/Create Measurements [Position]/Create Rotation Matrix /Create Skew Symmetric/Create 3x3 matrix ==
  a11 : Inport
  a12 : Inport  Port=2
  a13 : Inport  Port=3
  a21 : Inport  Port=4
  a22 : Inport  Port=5
  a23 : Inport  Port=6
  a31 : Inport  Port=7
  a32 : Inport  Port=8
  a33 : Inport  Port=9
  Math Function : Math  Operator=transpose  SaturateOnIntegerOverflow=on
  Reshape (9) to [3x3] column-major : Reshape  OutputDimensionality=Customize  OutputDimensions=[3,3]
  Vector Concatenate : Concatenate  NumInputs=9
  Matrix : Outport
  wires:
  Math Function/1 -> Matrix/1
  Reshape (9) to [3x3] column-major/1 -> Math Function/1
  a21/1 -> Vector Concatenate/4
  a32/1 -> Vector Concatenate/8
  a31/1 -> Vector Concatenate/7
  a23/1 -> Vector Concatenate/6
  a13/1 -> Vector Concatenate/3
  a12/1 -> Vector Concatenate/2
  a11/1 -> Vector Concatenate/1
  Vector Concatenate/1 -> Reshape (9) to [3x3] column-major/1
  a22/1 -> Vector Concatenate/5
  a33/1 -> Vector Concatenate/9

== system EKF_SIL_02_newdelIpsOOSM/Plots and display/Create Measurements [Pose]2/Create Measurements [Position]/Create Rotation Matrix 1/Create Skew Symmetric/Create 3x3 matrix ==
  a11 : Inport
  a12 : Inport  Port=2
  a13 : Inport  Port=3
  a21 : Inport  Port=4
  a22 : Inport  Port=5
  a23 : Inport  Port=6
  a31 : Inport  Port=7
  a32 : Inport  Port=8
  a33 : Inport  Port=9
  Math Function : Math  Operator=transpose  SaturateOnIntegerOverflow=on
  Reshape (9) to [3x3] column-major : Reshape  OutputDimensionality=Customize  OutputDimensions=[3,3]
  Vector Concatenate : Concatenate  NumInputs=9
  Matrix : Outport
  wires:
  Math Function/1 -> Matrix/1
  Reshape (9) to [3x3] column-major/1 -> Math Function/1
  a21/1 -> Vector Concatenate/4
  a32/1 -> Vector Concatenate/8
  a31/1 -> Vector Concatenate/7
  a23/1 -> Vector Concatenate/6
  a13/1 -> Vector Concatenate/3
  a12/1 -> Vector Concatenate/2
  a11/1 -> Vector Concatenate/1
  Vector Concatenate/1 -> Reshape (9) to [3x3] column-major/1
  a22/1 -> Vector Concatenate/5
  a33/1 -> Vector Concatenate/9

== system EKF_SIL_02_newdelIpsOOSM/EKF/Measurement Update/Update with K(k) and predict current state/Create H_k/Create Rotation Matrix /Create Skew Symmetric/Create 3x3 matrix ==
  a11 : Inport
  a12 : Inport  Port=2
  a13 : Inport  Port=3
  a21 : Inport  Port=4
  a22 : Inport  Port=5
  a23 : Inport  Port=6
  a31 : Inport  Port=7
  a32 : Inport  Port=8
  a33 : Inport  Port=9
  Math Function : Math  Operator=transpose  SaturateOnIntegerOverflow=on
  Reshape (9) to [3x3] column-major : Reshape  OutputDimensionality=Customize  OutputDimensions=[3,3]
  Vector Concatenate : Concatenate  NumInputs=9
  Matrix : Outport
  wires:
  a33/1 -> Vector Concatenate/9
  a22/1 -> Vector Concatenate/5
  Vector Concatenate/1 -> Reshape (9) to [3x3] column-major/1
  a11/1 -> Vector Concatenate/1
  a12/1 -> Vector Concatenate/2
  a13/1 -> Vector Concatenate/3
  a23/1 -> Vector Concatenate/6
  a31/1 -> Vector Concatenate/7
  a32/1 -> Vector Concatenate/8
  a21/1 -> Vector Concatenate/4
  Reshape (9) to [3x3] column-major/1 -> Math Function/1
  Math Function/1 -> Matrix/1

== system EKF_SIL_02_newdelIpsOOSM/EKF/Measurement Update/Update with K(k) and predict current state/Create H_k/Create Rotation Matrix 1/Create Skew Symmetric/Create 3x3 matrix ==
  a11 : Inport
  a12 : Inport  Port=2
  a13 : Inport  Port=3
  a21 : Inport  Port=4
  a22 : Inport  Port=5
  a23 : Inport  Port=6
  a31 : Inport  Port=7
  a32 : Inport  Port=8
  a33 : Inport  Port=9
  Math Function : Math  Operator=transpose  SaturateOnIntegerOverflow=on
  Reshape (9) to [3x3] column-major : Reshape  OutputDimensionality=Customize  OutputDimensions=[3,3]
  Vector Concatenate : Concatenate  NumInputs=9
  Matrix : Outport
  wires:
  Math Function/1 -> Matrix/1
  Reshape (9) to [3x3] column-major/1 -> Math Function/1
  a21/1 -> Vector Concatenate/4
  a32/1 -> Vector Concatenate/8
  a31/1 -> Vector Concatenate/7
  a23/1 -> Vector Concatenate/6
  a13/1 -> Vector Concatenate/3
  a12/1 -> Vector Concatenate/2
  a11/1 -> Vector Concatenate/1
  Vector Concatenate/1 -> Reshape (9) to [3x3] column-major/1
  a22/1 -> Vector Concatenate/5
  a33/1 -> Vector Concatenate/9

== system EKF_SIL_02_newdelIpsOOSM/EKF/Measurement Update/Update with K(k) and predict current state/Create H_k/Create Rotation Matrix 2/Create Skew Symmetric/Create 3x3 matrix ==
  a11 : Inport
  a12 : Inport  Port=2
  a13 : Inport  Port=3
  a21 : Inport  Port=4
  a22 : Inport  Port=5
  a23 : Inport  Port=6
  a31 : Inport  Port=7
  a32 : Inport  Port=8
  a33 : Inport  Port=9
  Math Function : Math  Operator=transpose  SaturateOnIntegerOverflow=on
  Reshape (9) to [3x3] column-major : Reshape  OutputDimensionality=Customize  OutputDimensions=[3,3]
  Vector Concatenate : Concatenate  NumInputs=9
  Matrix : Outport
  wires:
  a33/1 -> Vector Concatenate/9
  a22/1 -> Vector Concatenate/5
  Vector Concatenate/1 -> Reshape (9) to [3x3] column-major/1
  a11/1 -> Vector Concatenate/1
  a12/1 -> Vector Concatenate/2
  a13/1 -> Vector Concatenate/3
  a23/1 -> Vector Concatenate/6
  a31/1 -> Vector Concatenate/7
  a32/1 -> Vector Concatenate/8
  a21/1 -> Vector Concatenate/4
  Reshape (9) to [3x3] column-major/1 -> Math Function/1
  Math Function/1 -> Matrix/1

== system EKF_SIL_02_newdelIpsOOSM/EKF/Measurement Update/Update with K(k) and predict current state/Create h/Create Rotation Matrix /Create Skew Symmetric/Create 3x3 matrix ==
  a11 : Inport
  a12 : Inport  Port=2
  a13 : Inport  Port=3
  a21 : Inport  Port=4
  a22 : Inport  Port=5
  a23 : Inport  Port=6
  a31 : Inport  Port=7
  a32 : Inport  Port=8
  a33 : Inport  Port=9
  Math Function : Math  Operator=transpose  SaturateOnIntegerOverflow=on
  Reshape (9) to [3x3] column-major : Reshape  OutputDimensionality=Customize  OutputDimensions=[3,3]
  Vector Concatenate : Concatenate  NumInputs=9
  Matrix : Outport
  wires:
  a33/1 -> Vector Concatenate/9
  a22/1 -> Vector Concatenate/5
  Vector Concatenate/1 -> Reshape (9) to [3x3] column-major/1
  a11/1 -> Vector Concatenate/1
  a12/1 -> Vector Concatenate/2
  a13/1 -> Vector Concatenate/3
  a23/1 -> Vector Concatenate/6
  a31/1 -> Vector Concatenate/7
  a32/1 -> Vector Concatenate/8
  a21/1 -> Vector Concatenate/4
  Reshape (9) to [3x3] column-major/1 -> Math Function/1
  Math Function/1 -> Matrix/1

== system EKF_SIL_02_newdelIpsOOSM/EKF/Measurement Update/Update with K(k) and predict current state/Create h/Create Rotation Matrix 1/Create Skew Symmetric/Create 3x3 matrix ==
  a11 : Inport
  a12 : Inport  Port=2
  a13 : Inport  Port=3
  a21 : Inport  Port=4
  a22 : Inport  Port=5
  a23 : Inport  Port=6
  a31 : Inport  Port=7
  a32 : Inport  Port=8
  a33 : Inport  Port=9
  Math Function : Math  Operator=transpose  SaturateOnIntegerOverflow=on
  Reshape (9) to [3x3] column-major : Reshape  OutputDimensionality=Customize  OutputDimensions=[3,3]
  Vector Concatenate : Concatenate  NumInputs=9
  Matrix : Outport
  wires:
  a33/1 -> Vector Concatenate/9
  a22/1 -> Vector Concatenate/5
  Vector Concatenate/1 -> Reshape (9) to [3x3] column-major/1
  a11/1 -> Vector Concatenate/1
  a12/1 -> Vector Concatenate/2
  a13/1 -> Vector Concatenate/3
  a23/1 -> Vector Concatenate/6
  a31/1 -> Vector Concatenate/7
  a32/1 -> Vector Concatenate/8
  a21/1 -> Vector Concatenate/4
  Reshape (9) to [3x3] column-major/1 -> Math Function/1
  Math Function/1 -> Matrix/1

== system EKF_SIL_02_newdelIpsOOSM/EKF/Measurement Update/Update with K(k) and predict current state/Create h/Create Rotation Matrix 2/Create Skew Symmetric/Create 3x3 matrix ==
  a11 : Inport
  a12 : Inport  Port=2
  a13 : Inport  Port=3
  a21 : Inport  Port=4
  a22 : Inport  Port=5
  a23 : Inport  Port=6
  a31 : Inport  Port=7
  a32 : Inport  Port=8
  a33 : Inport  Port=9
  Math Function : Math  Operator=transpose  SaturateOnIntegerOverflow=on
  Reshape (9) to [3x3] column-major : Reshape  OutputDimensionality=Customize  OutputDimensions=[3,3]
  Vector Concatenate : Concatenate  NumInputs=9
  Matrix : Outport
  wires:
  Math Function/1 -> Matrix/1
  Reshape (9) to [3x3] column-major/1 -> Math Function/1
  a21/1 -> Vector Concatenate/4
  a32/1 -> Vector Concatenate/8
  a31/1 -> Vector Concatenate/7
  a23/1 -> Vector Concatenate/6
  a13/1 -> Vector Concatenate/3
  a12/1 -> Vector Concatenate/2
  a11/1 -> Vector Concatenate/1
  Vector Concatenate/1 -> Reshape (9) to [3x3] column-major/1
  a22/1 -> Vector Concatenate/5
  a33/1 -> Vector Concatenate/9

== system EKF_SIL_02_newdelIpsOOSM/EKF/OOSM_KF/OOSM_KF/State Propagation/Create Rotation Matrix 1/Create Skew Symmetric/Create 3x3 matrix ==
  a11 : Inport
  a12 : Inport  Port=2
  a13 : Inport  Port=3
  a21 : Inport  Port=4
  a22 : Inport  Port=5
  a23 : Inport  Port=6
  a31 : Inport  Port=7
  a32 : Inport  Port=8
  a33 : Inport  Port=9
  Math Function : Math  Operator=transpose  SaturateOnIntegerOverflow=on
  Reshape (9) to [3x3] column-major : Reshape  OutputDimensionality=Customize  OutputDimensions=[3,3]
  Vector Concatenate : Concatenate  NumInputs=9
  Matrix : Outport
  wires:
  a33/1 -> Vector Concatenate/9
  a22/1 -> Vector Concatenate/5
  Vector Concatenate/1 -> Reshape (9) to [3x3] column-major/1
  a11/1 -> Vector Concatenate/1
  a12/1 -> Vector Concatenate/2
  a13/1 -> Vector Concatenate/3
  a23/1 -> Vector Concatenate/6
  a31/1 -> Vector Concatenate/7
  a32/1 -> Vector Concatenate/8
  a21/1 -> Vector Concatenate/4
  Reshape (9) to [3x3] column-major/1 -> Math Function/1
  Math Function/1 -> Matrix/1

== system EKF_SIL_02_newdelIpsOOSM/EKF/OOSM_KF/OOSM_enable/Enabled Subsystem/Create H_k/Create Rotation Matrix /Create Skew Symmetric ==
  vector : Inport
  0 : Constant  Value=0
  Create 3x3 matrix : Subsystem
  Demux : Demux  Outputs=3
  Demux1 : Demux  Outputs=3
  Gain : Gain  Gain=-1
  skew symmetric Matrix : Outport
  wires:
  0/1 -> Create 3x3 matrix/1(a11), Create 3x3 matrix/9(a33), Create 3x3 matrix/5(a22)
  Demux/3 -> Create 3x3 matrix/2(a12)
  Demux1/2 -> Create 3x3 matrix/3(a13)
  Demux1/3 -> Create 3x3 matrix/4(a21)
  Demux/1 -> Create 3x3 matrix/6(a23)
  vector/1 -> Demux1/1, Gain/1
  Create 3x3 matrix/1(Matrix) -> skew symmetric Matrix/1
  Gain/1 -> Demux/1
  Demux/2 -> Create 3x3 matrix/7(a31)
  Demux1/1 -> Create 3x3 matrix/8(a32)

== system EKF_SIL_02_newdelIpsOOSM/EKF/OOSM_KF/OOSM_enable/Enabled Subsystem/Create H_k/Create Skew Symmetric/Create 3x3 matrix ==
  a11 : Inport
  a12 : Inport  Port=2
  a13 : Inport  Port=3
  a21 : Inport  Port=4
  a22 : Inport  Port=5
  a23 : Inport  Port=6
  a31 : Inport  Port=7
  a32 : Inport  Port=8
  a33 : Inport  Port=9
  Math Function : Math  Operator=transpose  SaturateOnIntegerOverflow=on
  Reshape (9) to [3x3] column-major : Reshape  OutputDimensionality=Customize  OutputDimensions=[3,3]
  Vector Concatenate : Concatenate  NumInputs=9
  Matrix : Outport
  wires:
  a33/1 -> Vector Concatenate/9
  a22/1 -> Vector Concatenate/5
  Vector Concatenate/1 -> Reshape (9) to [3x3] column-major/1
  a11/1 -> Vector Concatenate/1
  a12/1 -> Vector Concatenate/2
  a13/1 -> Vector Concatenate/3
  a23/1 -> Vector Concatenate/6
  a31/1 -> Vector Concatenate/7
  a32/1 -> Vector Concatenate/8
  a21/1 -> Vector Concatenate/4
  Reshape (9) to [3x3] column-major/1 -> Math Function/1
  Math Function/1 -> Matrix/1

== system EKF_SIL_02_newdelIpsOOSM/EKF/OOSM_KF/Subsystem/Dynamic Model (Differential equations)2/Dynamic Model (Differential equations)/Orbital Dynamics /Create Skew Symmetric ==
  vector : Inport
  0 : Constant  Value=0  SampleTime=-1
  Create 3x3 matrix : Subsystem
  Demux : Demux  Outputs=3
  Demux1 : Demux  Outputs=3
  Gain : Gain  Gain=-1
  skew symmetric Matrix : Outport
  wires:
  Demux1/1 -> Create 3x3 matrix/8(a32)
  Demux/2 -> Create 3x3 matrix/7(a31)
  Gain/1 -> Demux/1
  Create 3x3 matrix/1(Matrix) -> skew symmetric Matrix/1
  vector/1 -> Gain/1, Demux1/1
  Demux/1 -> Create 3x3 matrix/6(a23)
  Demux1/3 -> Create 3x3 matrix/4(a21)
  Demux1/2 -> Create 3x3 matrix/3(a13)
  Demux/3 -> Create 3x3 matrix/2(a12)
  0/1 -> Create 3x3 matrix/1(a11), Create 3x3 matrix/5(a22), Create 3x3 matrix/9(a33)

== system EKF_SIL_02_newdelIpsOOSM/EKF/OOSM_KF/Subsystem/Dynamic Model (Differential equations)2/Dynamic Model (Differential equations)/Orbital Dynamics /norm  ==
  vector : Inport
  Dot Product : DotProduct  InputSameDT=on  OutDataTypeStr=Inherit: Inherit via internal rule
  Sqrt : Sqrt  SaturateOnIntegerOverflow=on
  "norm " : Outport
  wires:
  Sqrt/1 -> "norm "/1
  vector/1 -> Dot Product/1, Dot Product/2
  Dot Product/1 -> Sqrt/1

== system EKF_SIL_02_newdelIpsOOSM/EKF/OOSM_KF/Subsystem/Dynamic Model (Differential equations)2/Dynamic Model (Differential equations)/Pose Servicer base//EE/Create Skew Symmetric ==
  vector : Inport
  0 : Constant  Value=0
  Create 3x3 matrix : Subsystem
  Demux : Demux  Outputs=3
  Demux1 : Demux  Outputs=3
  Gain : Gain  Gain=-1
  skew symmetric Matrix : Outport
  wires:
  0/1 -> Create 3x3 matrix/1(a11), Create 3x3 matrix/9(a33), Create 3x3 matrix/5(a22)
  Demux/3 -> Create 3x3 matrix/2(a12)
  Demux1/2 -> Create 3x3 matrix/3(a13)
  Demux1/3 -> Create 3x3 matrix/4(a21)
  Demux/1 -> Create 3x3 matrix/6(a23)
  vector/1 -> Demux1/1, Gain/1
  Create 3x3 matrix/1(Matrix) -> skew symmetric Matrix/1
  Gain/1 -> Demux/1
  Demux/2 -> Create 3x3 matrix/7(a31)
  Demux1/1 -> Create 3x3 matrix/8(a32)

== system EKF_SIL_02_newdelIpsOOSM/EKF/OOSM_KF/Subsystem/Dynamic Model (Differential equations)2/Dynamic Model (Differential equations)/Rotational Dynamics/Create  J ==
  p : Inport
  0 : Constant  Value=0  SampleTime=-1
  1 : Constant  SampleTime=-1
  Create 3x3 matrix : Subsystem
  Fcn : Fcn  Expr=1-u(2)/1+u(1)
  Fcn1 : Fcn  Expr=1+u(3)/1-u(1)
  "J_k " : Outport
  wires:
  1/1 -> Create 3x3 matrix/1(a11)
  Fcn1/1 -> Create 3x3 matrix/9(a33)
  Create 3x3 matrix/1(Matrix) -> "J_k "/1
  0/1 -> Create 3x3 matrix/2(a12), Create 3x3 matrix/3(a13), Create 3x3 matrix/4(a21), Create 3x3 matrix/6(a23), Create 3x3 matrix/7(a31), Create 3x3 matrix/8(a32)
  p/1 -> Fcn/1, Fcn1/1
  Fcn/1 -> Create 3x3 matrix/5(a22)

== system EKF_SIL_02_newdelIpsOOSM/EKF/OOSM_KF/Subsystem/Dynamic Model (Differential equations)2/Dynamic Model (Differential equations)/Rotational Dynamics/Create Psi ==
  "omega " : Inport
  p : Inport  Port=2
  Create Psi : Concatenate  NumInputs=3
  Demux : Demux  Outputs=3
  Demux1 : Demux  Outputs=3
  Product{,1..5} (6 alike) : Product
  Scope : Scope
      settings: SaveName=ScopeData20
  Psi : Outport
  wires:
  "omega "/1 -> Demux1/1
  Product3/1 -> Product2/2
  Product5/1 -> Product4/2
  Product1/1 -> Product/2
  Product/1 -> Create Psi/1
  Demux/2 -> Product2/1
  Create Psi/1 -> Psi/1, Scope/1
  Demux/1 -> Product/1
  Product2/1 -> Create Psi/2
  Demux1/2 -> Product5/1, Product1/1
  Demux1/1 -> Product3/1, Product5/2
  Product4/1 -> Create Psi/3
  Demux/3 -> Product4/1
  p/1 -> Demux/1
  Demux1/3 -> Product3/2, Product1/2

== system EKF_SIL_02_newdelIpsOOSM/EKF/Predictor/Create State error covariance (P)/State Propagation/Create Rotation Matrix 1/Create Skew Symmetric/Create 3x3 matrix ==
  a11 : Inport
  a12 : Inport  Port=2
  a13 : Inport  Port=3
  a21 : Inport  Port=4
  a22 : Inport  Port=5
  a23 : Inport  Port=6
  a31 : Inport  Port=7
  a32 : Inport  Port=8
  a33 : Inport  Port=9
  Math Function : Math  Operator=transpose  SaturateOnIntegerOverflow=on
  Reshape (9) to [3x3] column-major : Reshape  OutputDimensionality=Customize  OutputDimensions=[3,3]
  Vector Concatenate : Concatenate  NumInputs=9
  Matrix : Outport
  wires:
  a33/1 -> Vector Concatenate/9
  a22/1 -> Vector Concatenate/5
  Vector Concatenate/1 -> Reshape (9) to [3x3] column-major/1
  a11/1 -> Vector Concatenate/1
  a12/1 -> Vector Concatenate/2
  a13/1 -> Vector Concatenate/3
  a23/1 -> Vector Concatenate/6
  a31/1 -> Vector Concatenate/7
  a32/1 -> Vector Concatenate/8
  a21/1 -> Vector Concatenate/4
  Reshape (9) to [3x3] column-major/1 -> Math Function/1
  Math Function/1 -> Matrix/1

== system EKF_SIL_02_newdelIpsOOSM/EKF/Predictor/Integrator/Dynamic Model (Differential equations)2/Dynamic Model (Differential equations)/Orbital Dynamics /Create Skew Symmetric ==
  vector : Inport
  0 : Constant  Value=0  SampleTime=-1
  Create 3x3 matrix : Subsystem
  Demux : Demux  Outputs=3
  Demux1 : Demux  Outputs=3
  Gain : Gain  Gain=-1
  skew symmetric Matrix : Outport
  wires:
  Demux1/1 -> Create 3x3 matrix/8(a32)
  Demux/2 -> Create 3x3 matrix/7(a31)
  Gain/1 -> Demux/1
  Create 3x3 matrix/1(Matrix) -> skew symmetric Matrix/1
  vector/1 -> Gain/1, Demux1/1
  Demux/1 -> Create 3x3 matrix/6(a23)
  Demux1/3 -> Create 3x3 matrix/4(a21)
  Demux1/2 -> Create 3x3 matrix/3(a13)
  Demux/3 -> Create 3x3 matrix/2(a12)
  0/1 -> Create 3x3 matrix/1(a11), Create 3x3 matrix/5(a22), Create 3x3 matrix/9(a33)

== system EKF_SIL_02_newdelIpsOOSM/EKF/Predictor/Integrator/Dynamic Model (Differential equations)2/Dynamic Model (Differential equations)/Orbital Dynamics /norm  ==
  vector : Inport
  Dot Product : DotProduct  InputSameDT=on  OutDataTypeStr=Inherit: Inherit via internal rule
  Sqrt : Sqrt  SaturateOnIntegerOverflow=on
  "norm " : Outport
  wires:
  Sqrt/1 -> "norm "/1
  vector/1 -> Dot Product/1, Dot Product/2
  Dot Product/1 -> Sqrt/1

== system EKF_SIL_02_newdelIpsOOSM/EKF/Predictor/Integrator/Dynamic Model (Differential equations)2/Dynamic Model (Differential equations)/Pose Servicer base//EE/Create Skew Symmetric ==
  vector : Inport
  0 : Constant  Value=0
  Create 3x3 matrix : Subsystem
  Demux : Demux  Outputs=3
  Demux1 : Demux  Outputs=3
  Gain : Gain  Gain=-1
  skew symmetric Matrix : Outport
  wires:
  0/1 -> Create 3x3 matrix/1(a11), Create 3x3 matrix/9(a33), Create 3x3 matrix/5(a22)
  Demux/3 -> Create 3x3 matrix/2(a12)
  Demux1/2 -> Create 3x3 matrix/3(a13)
  Demux1/3 -> Create 3x3 matrix/4(a21)
  Demux/1 -> Create 3x3 matrix/6(a23)
  vector/1 -> Demux1/1, Gain/1
  Create 3x3 matrix/1(Matrix) -> skew symmetric Matrix/1
  Gain/1 -> Demux/1
  Demux/2 -> Create 3x3 matrix/7(a31)
  Demux1/1 -> Create 3x3 matrix/8(a32)

== system EKF_SIL_02_newdelIpsOOSM/EKF/Predictor/Integrator/Dynamic Model (Differential equations)2/Dynamic Model (Differential equations)/Rotational Dynamics/Create  J ==
  p : Inport
  0 : Constant  Value=0  SampleTime=-1
  1 : Constant  SampleTime=-1
  Create 3x3 matrix : Subsystem
  Fcn : Fcn  Expr=1-u(2)/1+u(1)
  Fcn1 : Fcn  Expr=1+u(3)/1-u(1)
  "J_k " : Outport
  wires:
  1/1 -> Create 3x3 matrix/1(a11)
  Fcn1/1 -> Create 3x3 matrix/9(a33)
  Create 3x3 matrix/1(Matrix) -> "J_k "/1
  0/1 -> Create 3x3 matrix/2(a12), Create 3x3 matrix/3(a13), Create 3x3 matrix/4(a21), Create 3x3 matrix/6(a23), Create 3x3 matrix/7(a31), Create 3x3 matrix/8(a32)
  p/1 -> Fcn/1, Fcn1/1
  Fcn/1 -> Create 3x3 matrix/5(a22)

== system EKF_SIL_02_newdelIpsOOSM/EKF/Predictor/Integrator/Dynamic Model (Differential equations)2/Dynamic Model (Differential equations)/Rotational Dynamics/Create Psi ==
  "omega " : Inport
  p : Inport  Port=2
  Create Psi : Concatenate  NumInputs=3
  Demux : Demux  Outputs=3
  Demux1 : Demux  Outputs=3
  Product{,1..5} (6 alike) : Product
  Scope : Scope
      settings: SaveName=ScopeData20
  Psi : Outport
  wires:
  "omega "/1 -> Demux1/1
  Product3/1 -> Product2/2
  Product5/1 -> Product4/2
  Product1/1 -> Product/2
  Product/1 -> Create Psi/1
  Demux/2 -> Product2/1
  Create Psi/1 -> Psi/1, Scope/1
  Demux/1 -> Product/1
  Product2/1 -> Create Psi/2
  Demux1/2 -> Product5/1, Product1/1
  Demux1/1 -> Product3/1, Product5/2
  Product4/1 -> Create Psi/3
  Demux/3 -> Product4/1
  p/1 -> Demux/1
  Demux1/3 -> Product3/2, Product1/2

== system EKF_SIL_02_newdelIpsOOSM/EKF/OOSM_KF/OOSM_enable/Enabled Subsystem/Create H_k/Create Rotation Matrix /Create Skew Symmetric/Create 3x3 matrix ==
  a11 : Inport
  a12 : Inport  Port=2
  a13 : Inport  Port=3
  a21 : Inport  Port=4
  a22 : Inport  Port=5
  a23 : Inport  Port=6
  a31 : Inport  Port=7
  a32 : Inport  Port=8
  a33 : Inport  Port=9
  Math Function : Math  Operator=transpose  SaturateOnIntegerOverflow=on
  Reshape (9) to [3x3] column-major : Reshape  OutputDimensionality=Customize  OutputDimensions=[3,3]
  Vector Concatenate : Concatenate  NumInputs=9
  Matrix : Outport
  wires:
  a33/1 -> Vector Concatenate/9
  a22/1 -> Vector Concatenate/5
  Vector Concatenate/1 -> Reshape (9) to [3x3] column-major/1
  a11/1 -> Vector Concatenate/1
  a12/1 -> Vector Concatenate/2
  a13/1 -> Vector Concatenate/3
  a23/1 -> Vector Concatenate/6
  a31/1 -> Vector Concatenate/7
  a32/1 -> Vector Concatenate/8
  a21/1 -> Vector Concatenate/4
  Reshape (9) to [3x3] column-major/1 -> Math Function/1
  Math Function/1 -> Matrix/1

== system EKF_SIL_02_newdelIpsOOSM/EKF/OOSM_KF/Subsystem/Dynamic Model (Differential equations)2/Dynamic Model (Differential equations)/Orbital Dynamics /Create Skew Symmetric/Create 3x3 matrix ==
  a11 : Inport
  a12 : Inport  Port=2
  a13 : Inport  Port=3
  a21 : Inport  Port=4
  a22 : Inport  Port=5
  a23 : Inport  Port=6
  a31 : Inport  Port=7
  a32 : Inport  Port=8
  a33 : Inport  Port=9
  Math Function : Math  Operator=transpose  SaturateOnIntegerOverflow=on
  Reshape (9) to [3x3] column-major : Reshape  OutputDimensionality=Customize  OutputDimensions=[3,3]
  Vector Concatenate : Concatenate  NumInputs=9
  Matrix : Outport
  wires:
  a33/1 -> Vector Concatenate/9
  a22/1 -> Vector Concatenate/5
  Vector Concatenate/1 -> Reshape (9) to [3x3] column-major/1
  a11/1 -> Vector Concatenate/1
  a12/1 -> Vector Concatenate/2
  a13/1 -> Vector Concatenate/3
  a23/1 -> Vector Concatenate/6
  a31/1 -> Vector Concatenate/7
  a32/1 -> Vector Concatenate/8
  a21/1 -> Vector Concatenate/4
  Reshape (9) to [3x3] column-major/1 -> Math Function/1
  Math Function/1 -> Matrix/1
